simulink model "AOO_example"  (R2020a)
settings: Solver=FixedStepAuto  StartTime=0.0  StopTime=10.0  FixedStep=1e-3  RelTol=1e-3  EnableMultiTasking=on
undefined symbols (not defined in the file): D10, D11, D2, D4, D5, D8, PTA0, PTA2, PTB23, PTB9, PTD0, PTD2
libraries: frdmk64flib x8
settings Model: ExtModeTrigDuration=5  Creator=tj200  LastModifiedBy=karir
settings OptimizationCC: EnhancedBackFolding=on  PassReuseOutputArgsAs=Individual arguments  ZeroExternalMemoryAtStartup=off  ZeroInternalMemoryAtStartup=off  MaxStackSize=64  OptimizeBlockOrder=speed  DifferentSizesBufferReuse=on  OptimizationCustomize=off  EfficientTunableParamExpr=on
settings DebuggingCC: ParameterTunabilityLossMsg=error
settings HardwareCC: ProdBitPerPointer=32  ProdBitPerSizeT=32  ProdBitPerPtrDiffT=32  ProdLargestAtomicInteger=Long  ProdLargestAtomicFloat=Double  ProdWordSize=32  ProdHWDeviceType=ARM Compatible->ARM Cortex
settings SFSimCC: MATLABDynamicMemAlloc=off
settings RTWCC: SystemTargetFile=ert.tlc  HardwareBoard=NXP FRDM-K64F  TemplateMakefile=ert_default_tmf  Toolchain=GNU Tools for ARM Embedded Processors
settings CodeAppCC: ForceParamTrailComments=on  IgnoreCustomStorageClasses=off  OperatorAnnotations=on  SimulinkDataObjDesc=on  SFDataObjDesc=on  InsertBlockDesc=on

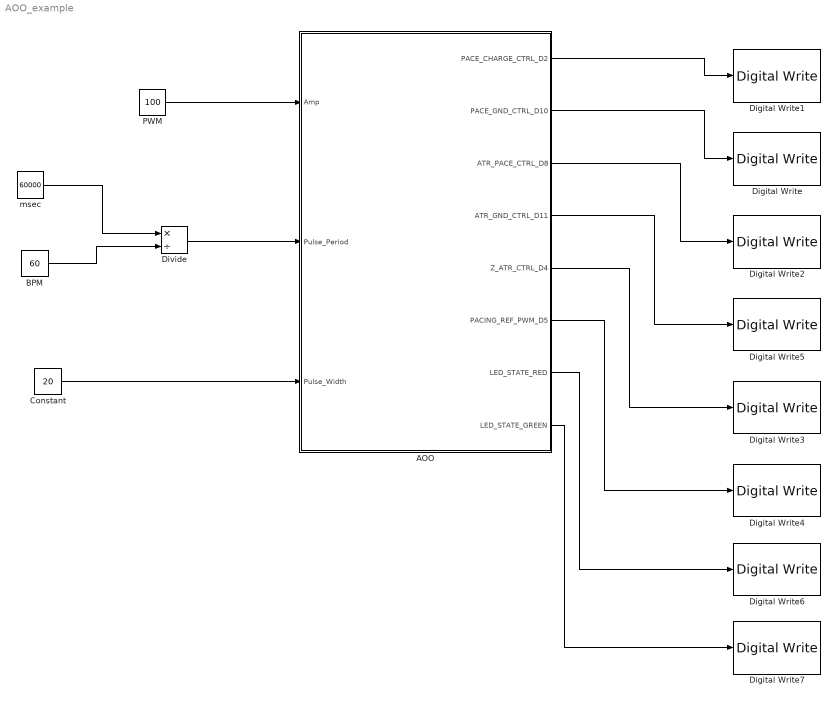
== system AOO_example ==
  AOO : Stateflow chart  TreatAsAtomicUnit=on
  BPM : Constant  Value=60
  Constant : Constant  Value=20
  Digital Write : frdmk64flib/Digital Write  Whichpin=PTD0 (D10)
  Digital Write1 : frdmk64flib/Digital Write  Whichpin=PTB9 (D2)
  Digital Write2 : frdmk64flib/Digital Write  Whichpin=PTA0 (D8)
  Digital Write3 : frdmk64flib/Digital Write  Whichpin=PTB23 (D4)
  Digital Write4 : frdmk64flib/Digital Write  Whichpin=PTA2 (D5)
  Digital Write5 : frdmk64flib/Digital Write  Whichpin=PTD2 (D11)
  Digital Write6 : frdmk64flib/Digital Write  Whichpin=RED_LED
  Digital Write7 : frdmk64flib/Digital Write  Whichpin=GREEN_LED
  Divide : Product  Inputs=*/
  PWM : Constant  Value=100
  msec : Constant  Value=60000
  wires:
  AOO/1(PACE_CHARGE_CTRL_D2) -> Digital Write1/1
  AOO/2(PACE_GND_CTRL_D10) -> Digital Write/1
  AOO/3(ATR_PACE_CTRL_D8) -> Digital Write2/1
  AOO/4(ATR_GND_CTRL_D11) -> Digital Write5/1
  PWM/1 -> AOO/1(Amp)
  AOO/6(PACING_REF_PWM_D5) -> Digital Write4/1
  AOO/5(Z_ATR_CTRL_D4) -> Digital Write3/1
  AOO/7(LED_STATE_RED) -> Digital Write6/1
  AOO/8(LED_STATE_GREEN) -> Digital Write7/1
  msec/1 -> Divide/1
  BPM/1 -> Divide/2
  Divide/1 -> AOO/2(Pulse_Period)
  Constant/1 -> AOO/3(Pulse_Width)

== stateflow chart AOO_example/AOO ==
  state pacing
    entry:
    PACING_REF_PWM_D5 = Amp;
    PACE_CHARGE_CTRL_D2=0;
    ATR_PACE_CTRL_D8= 1;
    ATR_GND_CTRL_D11= 0;
    PACE_GND_CTRL_D10=1;
    Z_ATR_CTRL_D4=0;
    LED_STATE_RED=false;
    LED_STATE_GREEN=true;
  state Chambers_Paced_Charging
    entry:
    PACING_REF_PWM_D5 = Amp;
    PACE_CHARGE_CTRL_D2=1;
    ATR_PACE_CTRL_D8= 0;
    ATR_GND_CTRL_D11= 1;
    PACE_GND_CTRL_D10=0;
    Z_ATR_CTRL_D4=0;
    LED_STATE_RED=true;
    LED_STATE_GREEN=false;
  (default) -> Chambers_Paced_Charging
  Chambers_Paced_Charging -> pacing : [after(Pulse_Period-Pulse_Width,msec)]
  pacing -> Chambers_Paced_Charging : [after(Pulse_Width,msec)]
  data: A_Atrium local; V_Ventricle local; I_Inhibited local; O_None local; ATR_CMP_DETECT_D0 local; VENT_CMP_DETECT_D1 local; VENT_CMP_REF_PWM_D3 local; ATR_CMP_REF_PWM_D6 local; Z_VENT_CTRL_D7 local; VENT_PACE_CTRL_D9 local; VENT_GND_CTRL_D12 local; FRONTEND_CTRL_D13 local; GND local; VENT_RECT_SIGNAL_A4_SDA local; ATR_RECT_SIGNAL_A3 local; Z_SIGNAL_A2 local; VENT_SIGNAL_A1 local; ATR_SIGNAL_A0 local; PACE_CHARGE_CTRL_D2 output; PACE_GND_CTRL_D10 output; ATR_PACE_CTRL_D8 output; ATR_GND_CTRL_D11 output; Z_ATR_CTRL_D4 output; PACING_REF_PWM_D5 output; Amp input; LED_STATE_RED output; LED_STATE_GREEN output; Pulse_Period input; Pulse_Width input
